simulink model "Complete_Vehicle_Model_qss"  (R2019a)
settings: Solver=VariableStepAuto  StartTime=0.0  StopTime=1220  RelTol=1e-3
undefined symbols (not defined in the file): DiscIntNeverNeededParam
libraries: qss_tb_library x6
settings Model: Creator=Sai_Mj  LastModifiedBy=Sai_Mj

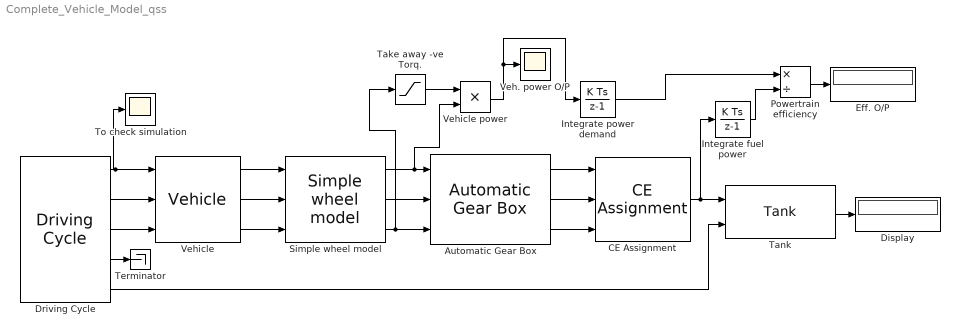
== system Complete_Vehicle_Model_qss ==
  "Automatic Gear Box " : qss_tb_library/Gear System/Automatic Gear Box  Tag=transmission  nog=5  i=[3.38 1.76 1.12 0.89 0.7]  i_diff=4.45  gearon=[10 25 40 70]  gearoff=[2 15 30 50]  d=0.62  e_GT=0.98  P_GT0=300  w_wheel_min=1
  "CE Assignment " : qss_tb_library/Energy Converter/CE Assignment  Tag=combustion engine  engine_type=Gasoline  P_ice=95  ENABLE_FUEL_CUTOFF=off
  "Display " : Display
  "Driving Cycle " : qss_tb_library/Driving Cycle/Driving Cycle  Tag=cycle  cyclename1=NEDC  stepsize=1  autostop=on
  "Eff. O/P " : Display
  "Integrate fuel power " : DiscreteIntegrator  SampleTime=-1  ICPrevOutput=DiscIntNeverNeededParam  ICPrevScaledInput=DiscIntNeverNeededParam
  "Integrate power demand " : DiscreteIntegrator  SampleTime=-1  ICPrevOutput=DiscIntNeverNeededParam  ICPrevScaledInput=DiscIntNeverNeededParam
  "Powertrain efficiency " : Product  Inputs=*/
  "Simple wheel model " : qss_tb_library/Vehicle/Simple wheel model  Tag=simple transmission  d_wheel=0.62
  "Take away -ve Torq. " : Saturate  UpperLimit=100000  LowerLimit=0
  "Tank " : qss_tb_library/Energy Source/Tank  Tag=tank  fuel=Gasoline  flag_cold_start=on
  "Terminator " : Terminator
  "To check simulation " : Scope
  "Veh. power O/P " : Scope
  "Vehicle " : qss_tb_library/Vehicle/Vehicle  Tag=vehicle  m_f=1295+80+100  A_f=2  cw=0.30  mu=0.013  k_inertia=4
  "Vehicle power " : Product
  wires:
  "Simple wheel model "/1 -> "Vehicle power "/2, "Automatic Gear Box "/1
  "Simple wheel model "/2 -> "Automatic Gear Box "/2
  "Simple wheel model "/3 -> "Take away -ve Torq. "/1, "Automatic Gear Box "/3
  "Vehicle "/1 -> "Simple wheel model "/1
  "Vehicle "/2 -> "Simple wheel model "/2
  "Vehicle "/3 -> "Simple wheel model "/3
  "Driving Cycle "/2 -> "Vehicle "/2
  "Driving Cycle "/3 -> "Vehicle "/3
  "Automatic Gear Box "/1 -> "CE Assignment "/1
  "Automatic Gear Box "/2 -> "CE Assignment "/2
  "Automatic Gear Box "/3 -> "CE Assignment "/3
  "CE Assignment "/1 -> "Integrate fuel power "/1, "Tank "/1
  "Tank "/1 -> "Display "/1
  "Driving Cycle "/5 -> "Tank "/2
  "Driving Cycle "/4 -> "Terminator "/1
  "Driving Cycle "/1 -> "Vehicle "/1, "To check simulation "/1
  "Take away -ve Torq. "/1 -> "Vehicle power "/1
  "Vehicle power "/1 -> "Veh. power O/P "/1, "Integrate power demand "/1
  "Integrate power demand "/1 -> "Powertrain efficiency "/1
  "Integrate fuel power "/1 -> "Powertrain efficiency "/2
  "Powertrain efficiency "/1 -> "Eff. O/P "/1
